simulink model "RobotX_ss_acousticsSKIP_dock_odoa_refer_model1021"  (R2014a)
settings: Solver=FixedStepDiscrete  StartTime=0.0  StopTime=inf  FixedStep=.25  RelTol=1e-3
undefined symbols (not defined in the file): Com1, Com2, Com3, Com4, DiscIntNeverNeededParam, standard
libraries: xpcseriallib x42, slrtlib x8, simulink x7, speedgoatlib x2, speedgoatlib_IO102 x1
(part 7 of 18)

== matlab function RobotX_ss_acousticsSKIP_dock_odoa_refer_model1021/Main FSM/ODOA/SLAM1/Models for prediction/Model7/Dynamic Model ==
  data: F_surge input; F_sway input; Torque input; u input; surgeAccel output; v input; psi input; swayAccel output; yawAccel output
function [surgeAccel, swayAccel, yawAccel] = ...
    WAM_V_3DOF(F_surge, F_sway, Torque, u, v, psi)
%Written by Anderson Lebbad on August 12, 2014
%Last Edited:

%This function was heavily based off of Ariel Qu's Vel3DOF_IvanV1. It was
%rewritten for real-time use.

%This function will produce the transient output surge velocity of a
%linearized model of the USV. It is assumed that the vehicle is equivalent
%to two cylinders in the water.

%%%%%DEFINED VARIABLE%%%%%%
%
%   Xext = Thrust from motors
%   Next = Moment from motor
%   m = Mass of vehicle
%   Xudot = Added mass in surge direction
%   Yvdot = Added mass in sway direction
%   Nrdot = Added mass from yaw
%   xg = offset from center of gravity
%   rho = density of seawater
%   S = wetted surface area
%   R = Reynolds number
%   Cd = Coefficient of drag
%   Cdc = Coefficient of drag for sway
%   nu = Kinematic viscosity
%   L = Length overall
%   T = draft
%   B = beam
%   SA = Surface area of cylinder experiencing sway
%   Iz = moment of inertia about Z axis
%
%%%%%%

% Force/Mometns from thrusters & control surfaces...

tau = [F_surge; F_sway; Torque];

% Calculate yaw rate
persistent lastHeading
if isempty(lastHeading)
    lastHeading = psi;
end
%Sample time
ts = .1;

r = (psi - lastHeading)/ts;

% Velocity & Angular velocity vectors
vel = [u; v; 0];
omega = [0; 0; r];

%define variables
m = 145.7;         % Total mass [kg] - reduced from 102
rho = 1025.9;   % density of seawater [kg/m^3]
L = 3.91*0.85;  % Length on the waterline [m]
B = 0.426;       % Demihull beam [m]
T = B*0.2;        % Draft of the demihull [m]
p_bar = 1.0; % sidehull separation - from centerplane vessel to centerplane demihull
Iz = 262.181;    % Mass moment of inertia about z-axis [kg*m^2]
xg = 0;         % Body-Fixed coordinate system taken to be center of gravity
yg = 0;         % Symmetrical Vessel
Cd = 1.1;       % Drag coefficient for a lateral cylinder
LCG = 1.485;        % Need to know where LCG wrt stern

% Vector location of port and starboard hulls
r_port = [-LCG; -p_bar; 0];   
r_stbd = [-LCG; p_bar; 0];

% Port and starboard hull velocities
vel_port = vel + cross(omega,r_port);
vel_stbd = vel + cross(omega,r_stbd);

u_port = vel_port(1);
u_stbd = vel_stbd(1);

% Port and starboard state vectors
state_port = vel_port + omega;
state_stbd = vel_stbd + omega;

%% Added Mass
% Estimated for each hull, then multiplied by 2 to account for both hulls
Xudot = -0.05*m;

%Using strip theory to estimate added mass coefficients
Nrdot = -(4.75/2*pi*rho*p_bar*T^4 + pi*rho*T^2*((L - LCG)^3 + LCG^3)/3);
Nvdot = - pi*rho*T^2*((L - LCG)^2 - LCG^2)/2;

Yrdot = Nvdot;
Yvdot = -rho*pi*T^2*L;

% Multiply by 2:
Xudot = 2*Xudot;
Nrdot = 2*Nrdot;
Nvdot = 2*Nvdot;
Yrdot = 2*Yrdot;
Yvdot = 2*Yvdot;

%Calculate Coefficient of Drag for Sway from 1950 SNAME approximation
Cdc= 1.1 + 0.0045*L/T - 0.1*B/T + 0.016*(B/T)^2;
SA = 2*pi/4*T*L; %projected area of pontoon for two pontoons

%% Linear Drag Terms
%Total Speed
U = sqrt(u^2+v^2);

Xu = 0;
Yv = -0.5*rho*abs(v)*2*Cdc*SA; %20 was the last working number %from SNAME 1950, x2 for two cylinders
%Nr = -0.5*pi*rho*U*T^2*L^2;
Nr = -pi*rho*U*T^2*L^2*.065;
Nv = -pi*rho*U*T^2*L*.01;
Yr = pi*rho*U*T^2*L*0.2;  %from Newman approximation in Lewandowski

%% Nonlinear Drag Terms

% Drag and Moment due to drag on entire vessel - includes nonlinear and
% linear drag terms
D_port = 0.5*(0.44*u_port^3 - 0.01*u_port^2 + 19*u_port);     % Can assume that this equation also takes into account Xu - so set Xu=0
D_stbd = 0.5*(0.44*u_stbd^3 - 0.01*u_stbd^2 + 19*u_stbd);     % Can assume that this equation also takes into account Xu - so set Xu=0

tau_drag = [-(D_port + D_stbd); 0; (D_stbd - D_port)*p_bar];

Xuu = 0;

%% Maneuvering Coefficient Matrices
% Added Mass Matrix
M = [(m - Xudot)      0              0;...
    0               (m - Yvdot)     (m*xg - Yrdot);...
    0               (m*xg - Nvdot)  (Iz - Nrdot)];

%Centripetal and Added Mass Centripetal force matrices
% C_RB = [
%     0                  0                0
%     0                  0                0
%     0                  0                0
%     ];

% C_RB = [
%     0                  0                -m*(xg*r + v)
%     0                  0                -m*(yg*r - u)
%     m*(xg*r + v)       m*(yg*r - u)     0
%     ];

% C_A = -[ %negative originally
%     0                               0           0
%     0                               0           0
%     0                               0           0
%     ];

% Negating centripetal acceleration for test
C_RB = 0;
C_A = 0;

D = -[Xu  0   0;...
      0   Yv  Yr;...
      0   Nv  Nr];

% Nonlinear Drag Coefficients
D_N = -[Xuu*u   0                       0;...
        0       0                       0;...
        0       0                       0];
    
%% Calculate the port and starboard force vectors
tau_port = -(C_RB + C_A + D + D_N)*state_port;
tau_stbd = -(C_RB + C_A + D + D_N)*state_stbd;


%% Sum the force vectors
tau_tot = tau + tau_drag + tau_port + tau_stbd...
    + cross(r_port,[tau_port(1);tau_port(2);0]) + ...
    cross(r_stbd,[tau_stbd(1);tau_stbd(2);0]);

% Calculate the time derivative of the state vector

accel = M\tau_tot;

%% Separate output

surgeAccel = accel(1);
swayAccel = accel(2);
yawAccel = accel(3);

end

== matlab function RobotX_ss_acousticsSKIP_dock_odoa_refer_model1021/Main FSM/ODOA/Path/LLA to NED ==
  data: LLAs input; NEDout output; NED_origin input
function NEDout = LLA2NEDfun(LLAs,NED_origin)
%Written by Anderson Lebbad on September 20, 2014
%Last edited by:
%
%This function converts a target Latitude, Longitude, Altitude (LLA) point
%into North, East, Down (NED) coordinates

NED  = zeros(4,2);
for i=1:4
%First convert to earth centered, earth fixed frame
GoalECEF = lla2ecef([LLAs(i,:)*(pi/180), 0]');
%Then convert from ECEF to North East Down
GoalNEDvect = ecef2ned(NED_origin'*(pi/180),GoalECEF);
NED(i,:) = GoalNEDvect(1:2)';
end


%Order outputs for grid
Xord = sortrows(NED,1);
Yord = sortrows(NED,2);

BLfirst = ismember(Yord(3:4,:),Xord(3,:),'rows');
if sum(BLfirst) >= 1
    BL = Xord(3,:);
    BR = Xord(4,:);
else
    BL = Xord(4,:);
    BR = Xord(3,:);
end

TRthird = ismember(Yord(1:2,:),Xord(1,:),'rows');
if sum(TRthird) >= 1
    TR = Xord(1,:);
    TL = Xord(2,:);
else
    TR = Xord(2,:);
    TL = Xord(1,:);
end

NEDout = [BL; BR; TL; TR];

end

function x_ecef = lla2ecef(x_lla)
% LLE2ECEF: Converts from geodetic latitude, longitude, and altitude to earth-centered earth-fixed Cartesian coordinates
% INPUT: latitude phi (rad), longitude lambda (rad), altitude h (m)
% OUTPUT: [x, y, z]' (m) earth-centered earth-fixed Cartesian coordinates
    a = 6378137; % equatorial radius of ellipsoid (semi-major axis) (m)
    b = 6356752; % polar axis radius of ellipsoid (semi-minor axis) (m)

    phi = x_lla(1);
    lambda = x_lla(2);
    h = x_lla(3);
    
    % auxiliar quantities f, e, and N
    f = (a-b)/a;
    e = f*(2-f);
    N = a/sqrt(1-(e*sin(phi))^2);
    x_ecef = [(N+h)*cos(phi)*cos(lambda); (N+h)*cos(phi)*sin(lambda); (N*(1-e^2)+h)*sin(phi)];
end

function [x_ned] = ecef2ned(ned_lla, x_ecef)
% ECEF2NED Converts from earth-centered, earth-fixed Cartesian coordinates to tangent plane
% INPUT:
% 1) x_ecef=[x,y,z]' (m) earth-centered, earth-fixed Cartesian coordinates
% 2) ned_lla=[phi,lambda]' consiting of latitude phi (rad), longitude lambda (rad) of NED origin
% OUTPUT:
% 1) x_ned=[x,y,z]' (m) in NED coordinate system with the origin [phi,lambda]'

    phi = ned_lla(1);
    lambda = ned_lla(2);

    % transformation  matrix
    T = [-sin(phi)*cos(lambda) -sin(phi)*sin(lambda)  cos(phi)
         -sin(lambda)           cos(lambda)           0
          cos(phi)*cos(lambda)   cos(phi)*sin(lambda)  sin(phi)];

     x_ned = T*(x_ecef-lla2ecef([phi, lambda, 0]')); % convert to NED
     x_ned(3) = -x_ned(3);
end

== matlab function RobotX_ss_acousticsSKIP_dock_odoa_refer_model1021/Main FSM/ODOA/SLAM1/Models for prediction/Model1/Stbd Thruster Model ==
  data: stbdMP input; F_surge output; stbdAzimuth input; F_sway output; Torque output
function [F_surge,F_sway,Torque]  = StarBoardThruster(stbdMP,stbdAzimuth)
%Approximation for Starboard Force and Moment with the input motor power
%and azimuth angle of thruster

%Longitudinal distance from center of mass
longDist =1.007;           %m

%Axial distance from center of mass
axialDist=1.485;            %m

%% Piece-wise thrust calculation

if stbdMP <= -51.0119
    F = .9140*stbdMP + 40;
elseif stbdMP >= 26.8367
    F = 1.658*stbdMP - 41.01;
else
    F = .12987*stbdMP;
end

%% Force components
F_surge=F*cos(stbdAzimuth*pi/180);       %N
F_sway=F*sin(stbdAzimuth*pi/180);       %N

%% Torque calculation

Torque = -F_surge*longDist - F_sway*axialDist;   %N.m

end

== system RobotX_ss_acousticsSKIP_dock_odoa_refer_model1021/Main FSM/ODOA/GPS Move/Output Reassign ==
  Vaild : Inport
  Data : Inport  Port=2
  Sensors : Inport  Port=3
  Acoustic Active : Constant  Value=0
  Bus Creator2 : BusCreator  Inputs=3
  Bus Creator3 : BusCreator  Inputs=3
  Bus Creator5 : BusCreator  Inputs=2
  Constant3 : Constant  Value=0
  Lidar Mode : Constant  Value=0
  Outputs : Outport
  wires:
  Sensors/1 -> Bus Creator5/2  "Sensors"
  Bus Creator5/1 -> Outputs/1  "Output Signals"
  Vaild/1 -> Bus Creator2/1  "Valid"
  Constant3/1 -> Bus Creator2/2  "Control Mode"
  Data/1 -> Bus Creator2/3  "Data"
  Bus Creator2/1 -> Bus Creator3/1  "Navigation Outputs"
  Acoustic Active/1 -> Bus Creator3/2  "Acoustic Active"
  Lidar Mode/1 -> Bus Creator3/3  "Lidar Mode"
  Bus Creator3/1 -> Bus Creator5/1  "Outputs"

== system RobotX_ss_acousticsSKIP_dock_odoa_refer_model1021/Main FSM/ODOA/Path/Output Reassign ==
  Vaild : Inport
  Data : Inport  Port=2
  Sensors : Inport  Port=3
  Acoustic Active : Constant  Value=0
  Bus Creator2 : BusCreator  Inputs=3
  Bus Creator3 : BusCreator  Inputs=3
  Bus Creator5 : BusCreator  Inputs=2
  Constant3 : Constant  Value=0
  Lidar Mode : Constant  Value=0
  Outputs : Outport
  wires:
  Sensors/1 -> Bus Creator5/2  "Sensors"
  Bus Creator5/1 -> Outputs/1  "Output Signals"
  Vaild/1 -> Bus Creator2/1  "Valid"
  Constant3/1 -> Bus Creator2/2  "Control Mode"
  Data/1 -> Bus Creator2/3  "Data"
  Bus Creator2/1 -> Bus Creator3/1  "Navigation Outputs"
  Acoustic Active/1 -> Bus Creator3/2  "Acoustic Active"
  Lidar Mode/1 -> Bus Creator3/3  "Lidar Mode"
  Bus Creator3/1 -> Bus Creator5/1  "Outputs"

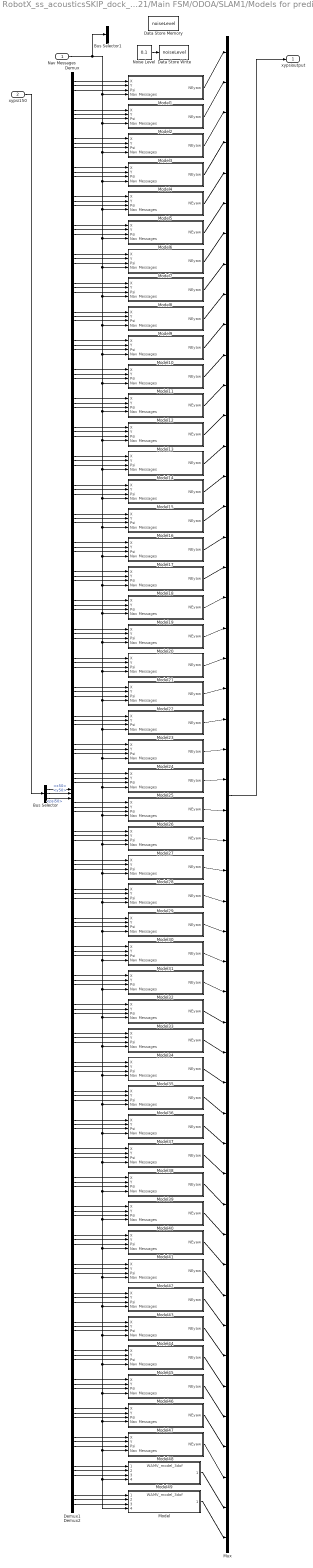
== system RobotX_ss_acousticsSKIP_dock_odoa_refer_model1021/Main FSM/ODOA/SLAM1/Models for prediction ==
  Nav Messages : Inport
  xypsi150 : Inport  Port=2
  Bus Selector : BusSelector  OutputSignals=x50,y50,psi50
  Bus Selector1 : BusSelector  OutputSignals=signal1,signal2
  Data Store Memory : DataStoreMemory  DataStoreName=noiseLevel  ReadBeforeWriteMsg=warning  WriteAfterWriteMsg=warning  WriteAfterReadMsg=warning
  Data Store Write : DataStoreWrite  DataStoreName=noiseLevel
  Demux : Demux  Outputs=50
  Demux1 : Demux  Outputs=50
  Demux2 : Demux  Outputs=50
  Model : ModelReference  ModelNameDialog=WAMV_model_3dof.slx  SimulationMode=Normal  ModelReferenceVersion=1.1919  CopyOfModelName=WAMV_model_3dof.slx  DefaultDataLogging=on
  Model1 : Subsystem
  Model10 : Subsystem
  Model11 : Subsystem
  Model12 : Subsystem
  Model13 : Subsystem
  Model14 : Subsystem
  Model15 : Subsystem
  Model16 : Subsystem
  Model17 : Subsystem
  Model18 : Subsystem
  Model19 : Subsystem
  Model2 : Subsystem
  Model20 : Subsystem
  Model21 : Subsystem
  Model22 : Subsystem
  Model23 : Subsystem
  Model24 : Subsystem
  Model25 : Subsystem
  Model26 : Subsystem
  Model27 : Subsystem
  Model28 : Subsystem
  Model29 : Subsystem
  Model3 : Subsystem
  Model30 : Subsystem
  Model31 : Subsystem
  Model32 : Subsystem
  Model33 : Subsystem
  Model34 : Subsystem
  Model35 : Subsystem
  Model36 : Subsystem
  Model37 : Subsystem
  Model38 : Subsystem
  Model39 : Subsystem
  Model4 : Subsystem
  Model40 : Subsystem
  Model41 : Subsystem
  Model42 : Subsystem
  Model43 : Subsystem
  Model44 : Subsystem
  Model45 : Subsystem
  Model46 : Subsystem
  Model47 : Subsystem
  Model48 : Subsystem
  Model49 : ModelReference  ModelNameDialog=WAMV_model_3dof.slx  SimulationMode=Normal  ModelReferenceVersion=1.1919  CopyOfModelName=WAMV_model_3dof.slx  DefaultDataLogging=on
  Model5 : Subsystem
  Model6 : Subsystem
  Model7 : Subsystem
  Model8 : Subsystem
  Model9 : Subsystem
  Mux : Mux  Inputs=50
  Noise Level : Constant  Value=0.1
  xypsioutput : Outport  PortDimensions=150
  wires:
  Noise Level/1 -> Data Store Write/1
  Demux/1 -> Model1/1(X)
  Demux1/1 -> Model1/2(Y)
  Demux2/1 -> Model1/3(Psi)
  Demux/2 -> Model2/1(X)
  Demux1/2 -> Model2/2(Y)
  Demux2/2 -> Model2/3(Psi)
  Demux/3 -> Model3/1(X)
  Demux1/3 -> Model3/2(Y)
  Demux2/3 -> Model3/3(Psi)
  Demux/4 -> Model4/1(X)
  Demux1/4 -> Model4/2(Y)
  Demux2/4 -> Model4/3(Psi)
  Demux/5 -> Model5/1(X)
  Demux1/5 -> Model5/2(Y)
  Demux2/5 -> Model5/3(Psi)
  Demux/6 -> Model6/1(X)
  Demux1/6 -> Model6/2(Y)
  Demux2/6 -> Model6/3(Psi)
  Nav Messages/1 -> Bus Selector1/1, Model1/4(Nav Messages), Model2/4(Nav Messages), Model3/4(Nav Messages), Model4/4(Nav Messages), Model5/4(Nav Messages), Model6/4(Nav Messages), Model7/4(Nav Messages), Model8/4(Nav Messages), Model9/4(Nav Messages), Model10/4(Nav Messages), Model11/4(Nav Messages), Model12/4(Nav Messages), Model13/4(Nav Messages), Model14/4(Nav Messages), Model15/4(Nav Messages), Model16/4(Nav Messages), Model17/4(Nav Messages), Model18/4(Nav Messages), Model19/4(Nav Messages), Model20/4(Nav Messages), Model21/4(Nav Messages), Model22/4(Nav Messages), Model23/4(Nav Messages), Model24/4(Nav Messages), Model25/4(Nav Messages), Model26/4(Nav Messages), Model27/4(Nav Messages), Model28/4(Nav Messages), Model29/4(Nav Messages), Model30/4(Nav Messages), Model31/4(Nav Messages), Model32/4(Nav Messages), Model33/4(Nav Messages), Model34/4(Nav Messages), Model35/4(Nav Messages), Model36/4(Nav Messages), Model37/4(Nav Messages), Model38/4(Nav Messages), Model39/4(Nav Messages), Model40/4(Nav Messages), Model41/4(Nav Messages), Model42/4(Nav Messages), Model43/4(Nav Messages), Model44/4(Nav Messages), Model45/4(Nav Messages), Model46/4(Nav Messages), Model47/4(Nav Messages), Model48/4(Nav Messages), Model49/4, Model/4
  Demux2/15 -> Model15/3(Psi)
  Demux1/15 -> Model15/2(Y)
  Demux/15 -> Model15/1(X)
  Demux2/14 -> Model14/3(Psi)
  Demux1/14 -> Model14/2(Y)
  Demux/14 -> Model14/1(X)
  Demux2/13 -> Model13/3(Psi)
  Demux1/13 -> Model13/2(Y)
  Demux/13 -> Model13/1(X)
  Demux2/12 -> Model12/3(Psi)
  Demux1/12 -> Model12/2(Y)
  Demux/12 -> Model12/1(X)
  Demux2/11 -> Model11/3(Psi)
  Demux1/11 -> Model11/2(Y)
  Demux/11 -> Model11/1(X)
  Demux2/10 -> Model10/3(Psi)
  Demux1/10 -> Model10/2(Y)
  Demux/10 -> Model10/1(X)
  Demux2/9 -> Model9/3(Psi)
  Demux1/9 -> Model9/2(Y)
  Demux/9 -> Model9/1(X)
  Demux2/8 -> Model8/3(Psi)
  Demux1/8 -> Model8/2(Y)
  Demux/8 -> Model8/1(X)
  Demux2/7 -> Model7/3(Psi)
  Demux1/7 -> Model7/2(Y)
  Demux/7 -> Model7/1(X)
  Demux/16 -> Model16/1(X)
  Demux1/16 -> Model16/2(Y)
  Demux2/16 -> Model16/3(Psi)
  Demux/17 -> Model17/1(X)
  Demux1/17 -> Model17/2(Y)
  Demux2/17 -> Model17/3(Psi)
  Demux/18 -> Model18/1(X)
  Demux1/18 -> Model18/2(Y)
  Demux2/18 -> Model18/3(Psi)
  Demux/19 -> Model19/1(X)
  Demux1/19 -> Model19/2(Y)
  Demux2/19 -> Model19/3(Psi)
  Demux/20 -> Model20/1(X)
  Demux1/20 -> Model20/2(Y)
  Demux2/20 -> Model20/3(Psi)
  Demux/21 -> Model21/1(X)
  Demux1/21 -> Model21/2(Y)
  Demux2/21 -> Model21/3(Psi)
  Demux/22 -> Model22/1(X)
  Demux1/22 -> Model22/2(Y)
  Demux2/22 -> Model22/3(Psi)
  Demux/23 -> Model23/1(X)
  Demux1/23 -> Model23/2(Y)
  Demux2/23 -> Model23/3(Psi)
  Demux/24 -> Model24/1(X)
  Demux1/24 -> Model24/2(Y)
  Demux2/24 -> Model24/3(Psi)
  Demux/25 -> Model25/1(X)
  Demux1/25 -> Model25/2(Y)
  Demux2/25 -> Model25/3(Psi)
  Demux/26 -> Model26/1(X)
  Demux1/26 -> Model26/2(Y)
  Demux2/26 -> Model26/3(Psi)
  Demux/27 -> Model27/1(X)
  Demux1/27 -> Model27/2(Y)
  Demux2/27 -> Model27/3(Psi)
  Demux/28 -> Model28/1(X)
  Demux1/28 -> Model28/2(Y)
  Demux2/28 -> Model28/3(Psi)
  Demux/29 -> Model29/1(X)
  Demux1/29 -> Model29/2(Y)
  Demux2/29 -> Model29/3(Psi)
  Demux/30 -> Model30/1(X)
  Demux1/30 -> Model30/2(Y)
  Demux2/30 -> Model30/3(Psi)
  Demux/31 -> Model31/1(X)
  Demux1/31 -> Model31/2(Y)
  Demux2/31 -> Model31/3(Psi)
  Demux/32 -> Model32/1(X)
  Demux1/32 -> Model32/2(Y)
  Demux2/32 -> Model32/3(Psi)
  Demux/33 -> Model33/1(X)
  Demux1/33 -> Model33/2(Y)
  Demux2/33 -> Model33/3(Psi)
  Demux/34 -> Model34/1(X)
  Demux1/34 -> Model34/2(Y)
  Demux2/34 -> Model34/3(Psi)
  Demux/35 -> Model35/1(X)
  Demux1/35 -> Model35/2(Y)
  Demux2/35 -> Model35/3(Psi)
  Demux/36 -> Model36/1(X)
  Demux1/36 -> Model36/2(Y)
  Demux2/36 -> Model36/3(Psi)
  Demux/37 -> Model37/1(X)
  Demux1/37 -> Model37/2(Y)
  Demux2/37 -> Model37/3(Psi)
  Demux/38 -> Model38/1(X)
  Demux1/38 -> Model38/2(Y)
  Demux2/38 -> Model38/3(Psi)
  Demux/39 -> Model39/1(X)
  Demux1/39 -> Model39/2(Y)
  Demux2/39 -> Model39/3(Psi)
  Demux/40 -> Model40/1(X)
  Demux1/40 -> Model40/2(Y)
  Demux2/40 -> Model40/3(Psi)
  Demux/41 -> Model41/1(X)
  Demux1/41 -> Model41/2(Y)
  Demux2/41 -> Model41/3(Psi)
  Demux/42 -> Model42/1(X)
  Demux1/42 -> Model42/2(Y)
  Demux2/42 -> Model42/3(Psi)
  Demux/43 -> Model43/1(X)
  Demux1/43 -> Model43/2(Y)
  Demux2/43 -> Model43/3(Psi)
  Demux/44 -> Model44/1(X)
  Demux1/44 -> Model44/2(Y)
  Demux2/44 -> Model44/3(Psi)
  Demux/45 -> Model45/1(X)
  Demux1/45 -> Model45/2(Y)
  Demux2/45 -> Model45/3(Psi)
  Demux/46 -> Model46/1(X)
  Demux1/46 -> Model46/2(Y)
  Demux2/46 -> Model46/3(Psi)
  Demux/47 -> Model47/1(X)
  Demux1/47 -> Model47/2(Y)
  Demux2/47 -> Model47/3(Psi)
  Demux/48 -> Model48/1(X)
  Demux1/48 -> Model48/2(Y)
  Demux2/48 -> Model48/3(Psi)
  Demux/49 -> Model49/1
  Demux1/49 -> Model49/2
  Demux2/49 -> Model49/3
  Demux/50 -> Model/1
  Demux1/50 -> Model/2
  Demux2/50 -> Model/3
  xypsi150/1 -> Bus Selector/1
  Bus Selector/1 -> Demux/1  "<x50>"
  Bus Selector/2 -> Demux1/1  "<y50>"
  Bus Selector/3 -> Demux2/1  "<psi50>"
  Model27/1(NEyaw) -> Mux/27
  Model26/1(NEyaw) -> Mux/26
  Model25/1(NEyaw) -> Mux/25
  Model24/1(NEyaw) -> Mux/24
  Model28/1(NEyaw) -> Mux/28
  Model23/1(NEyaw) -> Mux/23
  Model21/1(NEyaw) -> Mux/21
  Model30/1(NEyaw) -> Mux/30
  Model29/1(NEyaw) -> Mux/29
  Model22/1(NEyaw) -> Mux/22
  Model40/1(NEyaw) -> Mux/40
  Model33/1(NEyaw) -> Mux/33
  Model36/1(NEyaw) -> Mux/36
  Model38/1(NEyaw) -> Mux/38
  Model37/1(NEyaw) -> Mux/37
  Model35/1(NEyaw) -> Mux/35
  Model39/1(NEyaw) -> Mux/39
  Model31/1(NEyaw) -> Mux/31
  Model32/1(NEyaw) -> Mux/32
  Model34/1(NEyaw) -> Mux/34
  Model2/1(NEyaw) -> Mux/2
  Model5/1(NEyaw) -> Mux/5
  Model3/1(NEyaw) -> Mux/3
  Model4/1(NEyaw) -> Mux/4
  Model19/1(NEyaw) -> Mux/19
  Model13/1(NEyaw) -> Mux/13
  Model14/1(NEyaw) -> Mux/14
  Model12/1(NEyaw) -> Mux/12
  Model16/1(NEyaw) -> Mux/16
  Model17/1(NEyaw) -> Mux/17
  Model18/1(NEyaw) -> Mux/18
  Model20/1(NEyaw) -> Mux/20
  Model11/1(NEyaw) -> Mux/11
  Model15/1(NEyaw) -> Mux/15
  Model10/1(NEyaw) -> Mux/10
  Model8/1(NEyaw) -> Mux/8
  Model9/1(NEyaw) -> Mux/9
  Model7/1(NEyaw) -> Mux/7
  Model6/1(NEyaw) -> Mux/6
  Model48/1(NEyaw) -> Mux/48
  Model42/1(NEyaw) -> Mux/42
  Model49/1 -> Mux/49
  Model47/1(NEyaw) -> Mux/47
  Model/1 -> Mux/50
  Model43/1(NEyaw) -> Mux/43
  Model45/1(NEyaw) -> Mux/45
  Model44/1(NEyaw) -> Mux/44
  Model46/1(NEyaw) -> Mux/46
  Model41/1(NEyaw) -> Mux/41
  Model1/1(NEyaw) -> Mux/1
  Mux/1 -> xypsioutput/1

== system RobotX_ss_acousticsSKIP_dock_odoa_refer_model1021/Main FSM/ODOA/SLAM1/SLAM enabled ==
  pre_past_positions : Inport
  lm_data : Inport  Port=2
  positionboat : Inport  Port=3
  Enable : EnablePort
  slammed : MATLAB Function  TreatAsAtomicUnit=on
  mpa : Outport
  part_positions : Outport  Port=2
  wires:
  lm_data/1 -> slammed/1(lm_data)
  pre_past_positions/1 -> slammed/2(pre_part_positions)
  slammed/1(mpa) -> mpa/1
  slammed/2(part_positions) -> part_positions/1
  positionboat/1 -> slammed/3(positionboat)

== system RobotX_ss_acousticsSKIP_dock_odoa_refer_model1021/Main FSM/ODOA/SLAM1/inputselection ==
  controlchange : Inport
  xypsi : Inport  Port=2
  Landmarkchange : Inport  Port=3
  part_positions : Inport  Port=4
  xypsi150 : Inport  Port=5
  Bus Creator : BusCreator  Inputs=3
  Delay{,1..4} (5 alike) : Delay  DelayLength=1  InitialCondition=0
  MATLAB Function : MATLAB Function  TreatAsAtomicUnit=on
  last particle positions : Outport
  wires:
  Delay/1 -> MATLAB Function/4(part_positions)
  Delay1/1 -> MATLAB Function/3(xypsi)
  Delay2/1 -> MATLAB Function/5(xypsi150)
  Delay4/1 -> MATLAB Function/1(Landmarkchange)
  Delay3/1 -> MATLAB Function/2(controlchange)
  controlchange/1 -> Delay3/1
  xypsi/1 -> Delay1/1
  part_positions/1 -> Delay/1
  Landmarkchange/1 -> Delay4/1
  xypsi150/1 -> Delay2/1
  MATLAB Function/2(y50) -> Bus Creator/2  "y50"
  MATLAB Function/3(psi50) -> Bus Creator/3  "psi50"
  MATLAB Function/1(x50) -> Bus Creator/1  "x50"
  Bus Creator/1 -> last particle positions/1  "last particle positions"

== system RobotX_ss_acousticsSKIP_dock_odoa_refer_model1021/Main FSM/Start//Speedgate/Aim/Output Heirarchy ==
  Data : Inport
  Sensors : Inport  Port=2
  Acoustic Active : Constant  Value=0
  Bus Creator2 : BusCreator  Inputs=3
  Bus Creator3 : BusCreator  Inputs=3
  Bus Creator5 : BusCreator  Inputs=2
  Constant : Constant
  Constant3 : Constant
  Lidar Mode : Constant
  Outputs : Outport
  wires:
  Sensors/1 -> Bus Creator5/2  "Sensors"
  Bus Creator5/1 -> Outputs/1  "Output Signals"
  Constant/1 -> Bus Creator2/1  "Valid"
  Constant3/1 -> Bus Creator2/2  "Control Mode"
  Data/1 -> Bus Creator2/3  "Data"
  Bus Creator2/1 -> Bus Creator3/1  "Navigation Outputs"
  Acoustic Active/1 -> Bus Creator3/2  "Acoustic Active"
  Lidar Mode/1 -> Bus Creator3/3  "Lidar Mode"
  Bus Creator3/1 -> Bus Creator5/1  "Outputs"

== system RobotX_ss_acousticsSKIP_dock_odoa_refer_model1021/Main FSM/Start//Speedgate/Dead Reckon/Output Reassign ==
  Vaild : Inport
  Data : Inport  Port=2
  Sensors : Inport  Port=3
  Acoustic Active : Constant  Value=0
  Bus Creator2 : BusCreator  Inputs=3
  Bus Creator3 : BusCreator  Inputs=3
  Bus Creator5 : BusCreator  Inputs=2
  Constant3 : Constant  Value=0
  Lidar Mode : Constant  Value=3
  Outputs : Outport
  wires:
  Sensors/1 -> Bus Creator5/2  "Sensors"
  Bus Creator5/1 -> Outputs/1  "Output Signals"
  Vaild/1 -> Bus Creator2/1  "Valid"
  Constant3/1 -> Bus Creator2/2  "Control Mode"
  Data/1 -> Bus Creator2/3  "Data"
  Bus Creator2/1 -> Bus Creator3/1  "Navigation Outputs"
  Acoustic Active/1 -> Bus Creator3/2  "Acoustic Active"
  Lidar Mode/1 -> Bus Creator3/3  "Lidar Mode"
  Bus Creator3/1 -> Bus Creator5/1  "Outputs"

== system RobotX_ss_acousticsSKIP_dock_odoa_refer_model1021/Main FSM/Start//Speedgate/GPS Move/Output Reassign ==
  Vaild : Inport
  Data : Inport  Port=2
  Sensors : Inport  Port=3
  Acoustic Active : Constant  Value=0
  Bus Creator2 : BusCreator  Inputs=3
  Bus Creator3 : BusCreator  Inputs=3
  Bus Creator5 : BusCreator  Inputs=2
  Constant3 : Constant  Value=0
  Lidar Mode : Constant  Value=0
  Outputs : Outport
  wires:
  Sensors/1 -> Bus Creator5/2  "Sensors"
  Bus Creator5/1 -> Outputs/1  "Output Signals"
  Vaild/1 -> Bus Creator2/1  "Valid"
  Constant3/1 -> Bus Creator2/2  "Control Mode"
  Data/1 -> Bus Creator2/3  "Data"
  Bus Creator2/1 -> Bus Creator3/1  "Navigation Outputs"
  Acoustic Active/1 -> Bus Creator3/2  "Acoustic Active"
  Lidar Mode/1 -> Bus Creator3/3  "Lidar Mode"
  Bus Creator3/1 -> Bus Creator5/1  "Outputs"

== system RobotX_ss_acousticsSKIP_dock_odoa_refer_model1021/Sensors/1021 Comms/Message Selector/HRT Message ==
  Parameters : Inport
  Time : Inport  Port=2
  Bus Selector : BusSelector  OutputSignals=Sensors.Navigation Message.GPS (LLA).Lat,Sensors.Navigation Message.GPS (LLA).Long,Sensors.Navigation Message.On/Off/RC/Auto,Main Task
  MATLAB Function : MATLAB Function  TreatAsAtomicUnit=on
  HRT Message : Outport
  wires:
  MATLAB Function/1(asciiHRT) -> HRT Message/1
  Parameters/1 -> Bus Selector/1
  Time/1 -> MATLAB Function/1(Time)
  Bus Selector/1 -> MATLAB Function/2(HRTLat)  "<Lat>"
  Bus Selector/2 -> MATLAB Function/3(HRTLong)  "<Long>"
  Bus Selector/3 -> MATLAB Function/4(HRTMode)  "<On/Off/RC/Auto>"
  Bus Selector/4 -> MATLAB Function/5(HRTTask)  "<Main Task>"

== system RobotX_ss_acousticsSKIP_dock_odoa_refer_model1021/Sensors/1021 Comms/Message Selector/HRTLIT Message ==
  Parameters : Inport
  Time : Inport  Port=2
  Bus Selector : BusSelector  OutputSignals=Sensors.Navigation Message.GPS (LLA).Lat,Sensors.Navigation Message.GPS (LLA).Long,Main Task,Sensors.Navigation Message.On/Off/RC/Auto
  Data Store Read1 : DataStoreRead  DataStoreName=ltSeq
  MATLAB Function : MATLAB Function  TreatAsAtomicUnit=on
  MATLAB Function1 : MATLAB Function  TreatAsAtomicUnit=on
  HRTLIT Message : Outport
  wires:
  MATLAB Function/1(asciiHRTLIT) -> HRTLIT Message/1
  Time/1 -> MATLAB Function/1(Time)
  Parameters/1 -> Bus Selector/1
  Bus Selector/3 -> MATLAB Function/4(HRTTask)  "<Main Task>"
  Bus Selector/2 -> MATLAB Function/3(HRTLong)  "<Long>"
  Bus Selector/1 -> MATLAB Function/2(HRTLat)  "<Lat>"
  Bus Selector/4 -> MATLAB Function/5(HRTMode)  "<On/Off/RC/Auto>"
  Data Store Read1/1 -> MATLAB Function1/1(ltSeq)
  MATLAB Function1/2(LITSequence) -> MATLAB Function/7(LITSequence)
  MATLAB Function1/1(LITValid) -> MATLAB Function/6(LITValid)

== system RobotX_ss_acousticsSKIP_dock_odoa_refer_model1021/Sensors/1021 Comms/Message Selector/HRTSEA Message ==
  Parameters : Inport
  Time : Inport  Port=2
  Bus Selector : BusSelector  OutputSignals=Sensors.Navigation Message.GPS (LLA).Lat,Sensors.Navigation Message.GPS (LLA).Long,Main Task,Sensors.Navigation Message.On/Off/RC/Auto
  Data Store Read3 : DataStoreRead  DataStoreName=pingerInfo
  MATLAB Function : MATLAB Function  TreatAsAtomicUnit=on
  MATLAB Function1 : MATLAB Function  TreatAsAtomicUnit=on
  HRTSEA Message : Outport
  wires:
  MATLAB Function/1(asciiHRTSEA) -> HRTSEA Message/1
  Parameters/1 -> Bus Selector/1
  Time/1 -> MATLAB Function/1(Time)
  Data Store Read3/1 -> MATLAB Function1/1(pingerInfo)
  Bus Selector/3 -> MATLAB Function/4(HRTTask)  "<Main Task>"
  Bus Selector/1 -> MATLAB Function/2(HRTLat)  "<Lat>"
  Bus Selector/2 -> MATLAB Function/3(HRTLong)  "<Long>"
  Bus Selector/4 -> MATLAB Function/5(HRTMode)  "<On/Off/RC/Auto>"
  MATLAB Function1/3(SEALong) -> MATLAB Function/8(SEALong)
  MATLAB Function1/2(SEALat) -> MATLAB Function/7(SEALat)
  MATLAB Function1/5(SEADepth) -> MATLAB Function/10(SEADepth)
  MATLAB Function1/4(SEAColor) -> MATLAB Function/9(SEAColor)
  MATLAB Function1/1(SEAValid) -> MATLAB Function/6(SEAValid)

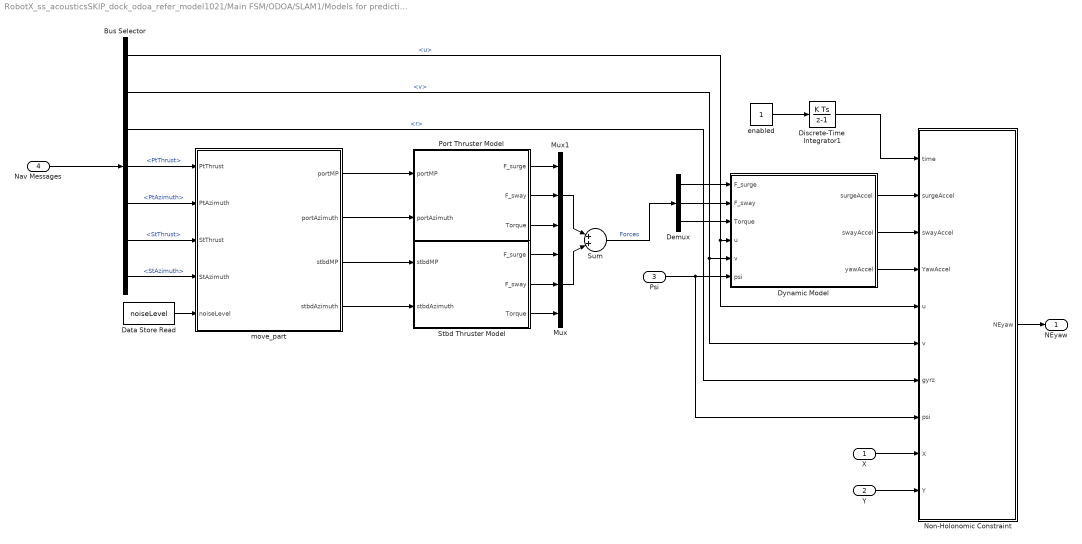
== system RobotX_ss_acousticsSKIP_dock_odoa_refer_model1021/Main FSM/ODOA/SLAM1/Models for prediction/Model1 ==
  X : Inport
  Y : Inport  Port=2
  Psi : Inport  Port=3
  Nav Messages : Inport  Port=4
  Bus Selector : BusSelector  OutputSignals=Velocity.u,Velocity.v,Velocity.r,Port.PtThrust,Port.PtAzimuth,Stbd.StThrust,Stbd.StAzimuth
  Data Store Read : DataStoreRead  DataStoreName=noiseLevel
  Demux : Demux  Outputs=3
  Discrete-Time Integrator1 : DiscreteIntegrator  SampleTime=-1  ICPrevOutput=DiscIntNeverNeededParam  ICPrevScaledInput=DiscIntNeverNeededParam
  Dynamic Model : MATLAB Function  TreatAsAtomicUnit=on
  Mux : Mux  Inputs=3
  Mux1 : Mux  Inputs=3
  Non-Holonomic Constraint : MATLAB Function  TreatAsAtomicUnit=on
  Port Thruster Model : MATLAB Function  TreatAsAtomicUnit=on
  Stbd Thruster Model : MATLAB Function  TreatAsAtomicUnit=on
  Sum : Sum  Inputs=|++|
  enabled : Constant
  move_part : MATLAB Function  TreatAsAtomicUnit=on
  NEyaw : Outport
  wires:
  Sum/1 -> Demux/1  "Forces"
  Bus Selector/2 -> Non-Holonomic Constraint/6(v), Dynamic Model/5(v)  "<v>"
  Bus Selector/1 -> Non-Holonomic Constraint/5(u), Dynamic Model/4(u)  "<u>"
  Psi/1 -> Non-Holonomic Constraint/8(psi), Dynamic Model/6(psi)
  Demux/2 -> Dynamic Model/2(F_sway)
  Demux/3 -> Dynamic Model/3(Torque)
  Demux/1 -> Dynamic Model/1(F_surge)
  Mux/1 -> Sum/2
  Stbd Thruster Model/1(F_surge) -> Mux/1
  Stbd Thruster Model/3(Torque) -> Mux/3
  Stbd Thruster Model/2(F_sway) -> Mux/2
  Mux1/1 -> Sum/1
  Port Thruster Model/2(F_sway) -> Mux1/2
  Port Thruster Model/1(F_surge) -> Mux1/1
  Port Thruster Model/3(Torque) -> Mux1/3
  Dynamic Model/1(surgeAccel) -> Non-Holonomic Constraint/2(surgeAccel)
  Dynamic Model/2(swayAccel) -> Non-Holonomic Constraint/3(swayAccel)
  Dynamic Model/3(yawAccel) -> Non-Holonomic Constraint/4(YawAccel)
  Y/1 -> Non-Holonomic Constraint/10(Y)
  X/1 -> Non-Holonomic Constraint/9(X)
  Bus Selector/3 -> Non-Holonomic Constraint/7(gyrz)  "<r>"
  Non-Holonomic Constraint/1(NEyaw) -> NEyaw/1
  enabled/1 -> Discrete-Time Integrator1/1
  Discrete-Time Integrator1/1 -> Non-Holonomic Constraint/1(time)
  Nav Messages/1 -> Bus Selector/1
  Bus Selector/4 -> move_part/1(PtThrust)  "<PtThrust>"
  Bus Selector/5 -> move_part/2(PtAzimuth)  "<PtAzimuth>"
  Bus Selector/7 -> move_part/4(StAzimuth)  "<StAzimuth>"
  Bus Selector/6 -> move_part/3(StThrust)  "<StThrust>"
  move_part/1(portMP) -> Port Thruster Model/1(portMP)
  move_part/2(portAzimuth) -> Port Thruster Model/2(portAzimuth)
  move_part/3(stbdMP) -> Stbd Thruster Model/1(stbdMP)
  move_part/4(stbdAzimuth) -> Stbd Thruster Model/2(stbdAzimuth)
  Data Store Read/1 -> move_part/5(noiseLevel)

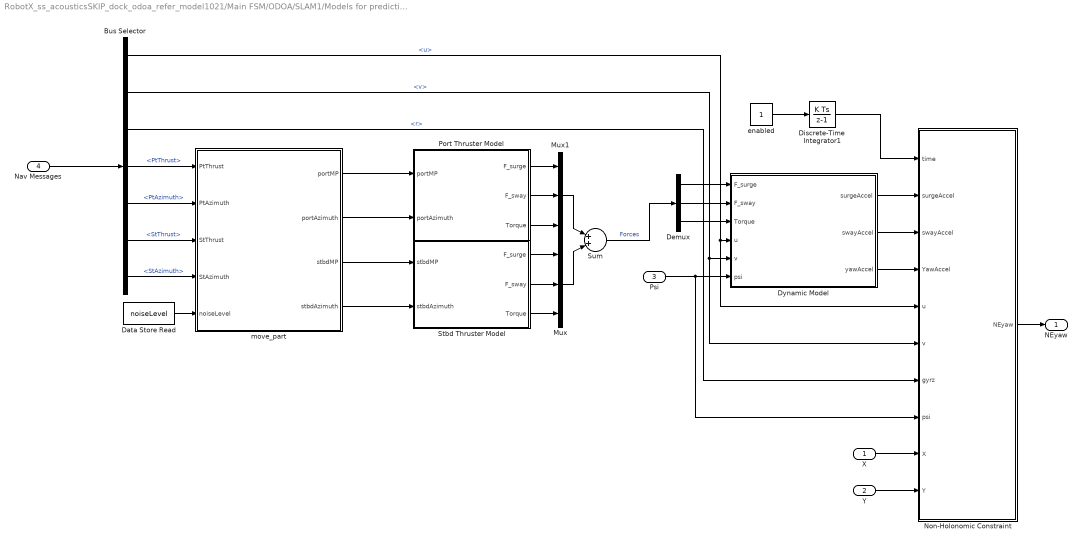
== system RobotX_ss_acousticsSKIP_dock_odoa_refer_model1021/Main FSM/ODOA/SLAM1/Models for prediction/Model10 ==
  X : Inport
  Y : Inport  Port=2
  Psi : Inport  Port=3
  Nav Messages : Inport  Port=4
  Bus Selector : BusSelector  OutputSignals=Velocity.u,Velocity.v,Velocity.r,Port.PtThrust,Port.PtAzimuth,Stbd.StThrust,Stbd.StAzimuth
  Data Store Read : DataStoreRead  DataStoreName=noiseLevel
  Demux : Demux  Outputs=3
  Discrete-Time Integrator1 : DiscreteIntegrator  SampleTime=-1  ICPrevOutput=DiscIntNeverNeededParam  ICPrevScaledInput=DiscIntNeverNeededParam
  Dynamic Model : MATLAB Function  TreatAsAtomicUnit=on
  Mux : Mux  Inputs=3
  Mux1 : Mux  Inputs=3
  Non-Holonomic Constraint : MATLAB Function  TreatAsAtomicUnit=on
  Port Thruster Model : MATLAB Function  TreatAsAtomicUnit=on
  Stbd Thruster Model : MATLAB Function  TreatAsAtomicUnit=on
  Sum : Sum  Inputs=|++|
  enabled : Constant
  move_part : MATLAB Function  TreatAsAtomicUnit=on
  NEyaw : Outport
  wires:
  Sum/1 -> Demux/1  "Forces"
  Bus Selector/2 -> Non-Holonomic Constraint/6(v), Dynamic Model/5(v)  "<v>"
  Bus Selector/1 -> Non-Holonomic Constraint/5(u), Dynamic Model/4(u)  "<u>"
  Psi/1 -> Non-Holonomic Constraint/8(psi), Dynamic Model/6(psi)
  Demux/2 -> Dynamic Model/2(F_sway)
  Demux/3 -> Dynamic Model/3(Torque)
  Demux/1 -> Dynamic Model/1(F_surge)
  Mux/1 -> Sum/2
  Stbd Thruster Model/1(F_surge) -> Mux/1
  Stbd Thruster Model/3(Torque) -> Mux/3
  Stbd Thruster Model/2(F_sway) -> Mux/2
  Mux1/1 -> Sum/1
  Port Thruster Model/2(F_sway) -> Mux1/2
  Port Thruster Model/1(F_surge) -> Mux1/1
  Port Thruster Model/3(Torque) -> Mux1/3
  Dynamic Model/1(surgeAccel) -> Non-Holonomic Constraint/2(surgeAccel)
  Dynamic Model/2(swayAccel) -> Non-Holonomic Constraint/3(swayAccel)
  Dynamic Model/3(yawAccel) -> Non-Holonomic Constraint/4(YawAccel)
  Y/1 -> Non-Holonomic Constraint/10(Y)
  X/1 -> Non-Holonomic Constraint/9(X)
  Bus Selector/3 -> Non-Holonomic Constraint/7(gyrz)  "<r>"
  Non-Holonomic Constraint/1(NEyaw) -> NEyaw/1
  enabled/1 -> Discrete-Time Integrator1/1
  Discrete-Time Integrator1/1 -> Non-Holonomic Constraint/1(time)
  Nav Messages/1 -> Bus Selector/1
  Bus Selector/4 -> move_part/1(PtThrust)  "<PtThrust>"
  Bus Selector/5 -> move_part/2(PtAzimuth)  "<PtAzimuth>"
  Bus Selector/7 -> move_part/4(StAzimuth)  "<StAzimuth>"
  Bus Selector/6 -> move_part/3(StThrust)  "<StThrust>"
  move_part/1(portMP) -> Port Thruster Model/1(portMP)
  move_part/2(portAzimuth) -> Port Thruster Model/2(portAzimuth)
  move_part/3(stbdMP) -> Stbd Thruster Model/1(stbdMP)
  move_part/4(stbdAzimuth) -> Stbd Thruster Model/2(stbdAzimuth)
  Data Store Read/1 -> move_part/5(noiseLevel)

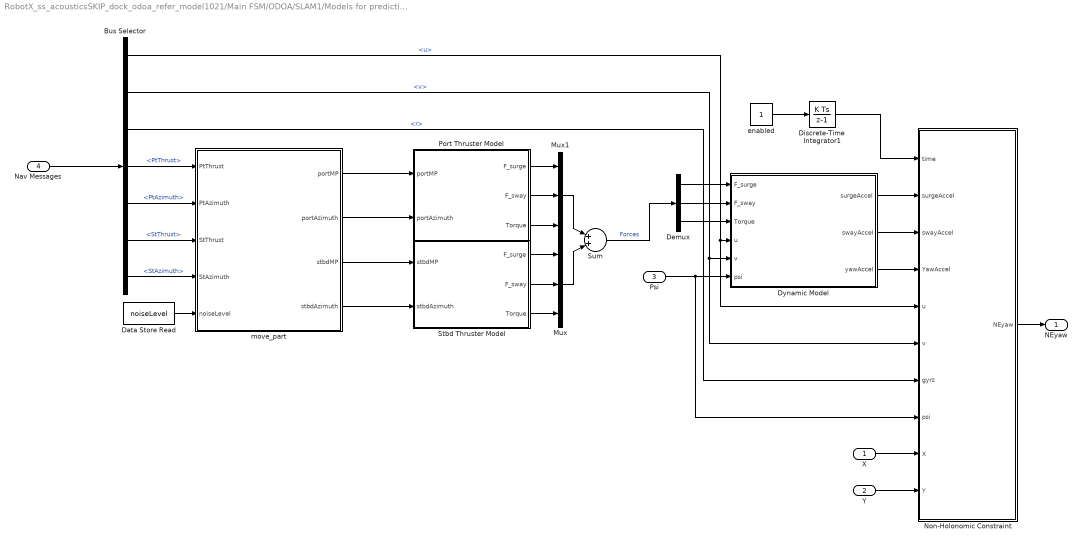
== system RobotX_ss_acousticsSKIP_dock_odoa_refer_model1021/Main FSM/ODOA/SLAM1/Models for prediction/Model11 ==
  X : Inport
  Y : Inport  Port=2
  Psi : Inport  Port=3
  Nav Messages : Inport  Port=4
  Bus Selector : BusSelector  OutputSignals=Velocity.u,Velocity.v,Velocity.r,Port.PtThrust,Port.PtAzimuth,Stbd.StThrust,Stbd.StAzimuth
  Data Store Read : DataStoreRead  DataStoreName=noiseLevel
  Demux : Demux  Outputs=3
  Discrete-Time Integrator1 : DiscreteIntegrator  SampleTime=-1  ICPrevOutput=DiscIntNeverNeededParam  ICPrevScaledInput=DiscIntNeverNeededParam
  Dynamic Model : MATLAB Function  TreatAsAtomicUnit=on
  Mux : Mux  Inputs=3
  Mux1 : Mux  Inputs=3
  Non-Holonomic Constraint : MATLAB Function  TreatAsAtomicUnit=on
  Port Thruster Model : MATLAB Function  TreatAsAtomicUnit=on
  Stbd Thruster Model : MATLAB Function  TreatAsAtomicUnit=on
  Sum : Sum  Inputs=|++|
  enabled : Constant
  move_part : MATLAB Function  TreatAsAtomicUnit=on
  NEyaw : Outport
  wires:
  Sum/1 -> Demux/1  "Forces"
  Bus Selector/2 -> Non-Holonomic Constraint/6(v), Dynamic Model/5(v)  "<v>"
  Bus Selector/1 -> Non-Holonomic Constraint/5(u), Dynamic Model/4(u)  "<u>"
  Psi/1 -> Non-Holonomic Constraint/8(psi), Dynamic Model/6(psi)
  Demux/2 -> Dynamic Model/2(F_sway)
  Demux/3 -> Dynamic Model/3(Torque)
  Demux/1 -> Dynamic Model/1(F_surge)
  Mux/1 -> Sum/2
  Stbd Thruster Model/1(F_surge) -> Mux/1
  Stbd Thruster Model/3(Torque) -> Mux/3
  Stbd Thruster Model/2(F_sway) -> Mux/2
  Mux1/1 -> Sum/1
  Port Thruster Model/2(F_sway) -> Mux1/2
  Port Thruster Model/1(F_surge) -> Mux1/1
  Port Thruster Model/3(Torque) -> Mux1/3
  Dynamic Model/1(surgeAccel) -> Non-Holonomic Constraint/2(surgeAccel)
  Dynamic Model/2(swayAccel) -> Non-Holonomic Constraint/3(swayAccel)
  Dynamic Model/3(yawAccel) -> Non-Holonomic Constraint/4(YawAccel)
  Y/1 -> Non-Holonomic Constraint/10(Y)
  X/1 -> Non-Holonomic Constraint/9(X)
  Bus Selector/3 -> Non-Holonomic Constraint/7(gyrz)  "<r>"
  Non-Holonomic Constraint/1(NEyaw) -> NEyaw/1
  enabled/1 -> Discrete-Time Integrator1/1
  Discrete-Time Integrator1/1 -> Non-Holonomic Constraint/1(time)
  Nav Messages/1 -> Bus Selector/1
  Bus Selector/4 -> move_part/1(PtThrust)  "<PtThrust>"
  Bus Selector/5 -> move_part/2(PtAzimuth)  "<PtAzimuth>"
  Bus Selector/7 -> move_part/4(StAzimuth)  "<StAzimuth>"
  Bus Selector/6 -> move_part/3(StThrust)  "<StThrust>"
  move_part/1(portMP) -> Port Thruster Model/1(portMP)
  move_part/2(portAzimuth) -> Port Thruster Model/2(portAzimuth)
  move_part/3(stbdMP) -> Stbd Thruster Model/1(stbdMP)
  move_part/4(stbdAzimuth) -> Stbd Thruster Model/2(stbdAzimuth)
  Data Store Read/1 -> move_part/5(noiseLevel)

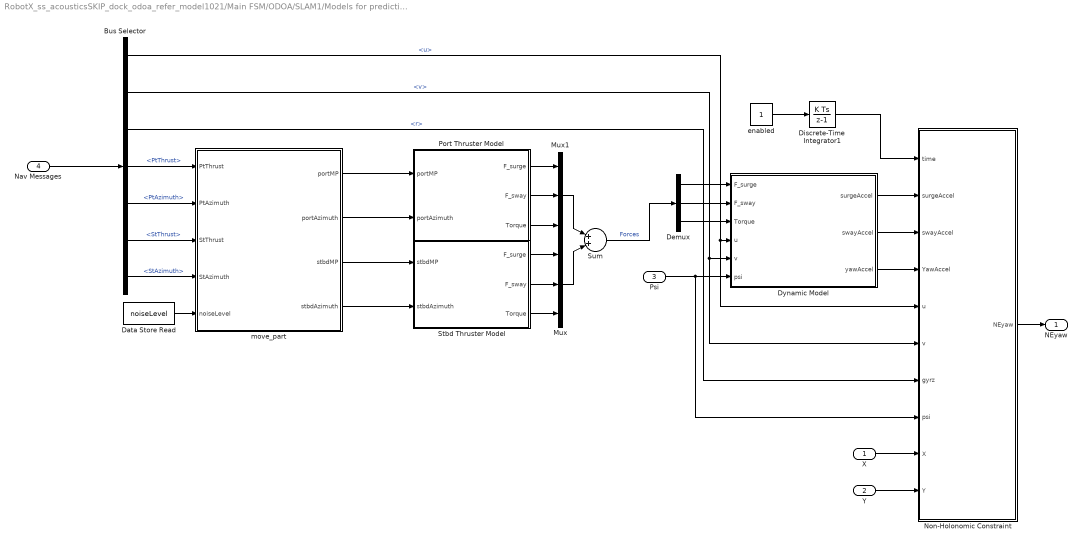
== system RobotX_ss_acousticsSKIP_dock_odoa_refer_model1021/Main FSM/ODOA/SLAM1/Models for prediction/Model12 ==
  X : Inport
  Y : Inport  Port=2
  Psi : Inport  Port=3
  Nav Messages : Inport  Port=4
  Bus Selector : BusSelector  OutputSignals=Velocity.u,Velocity.v,Velocity.r,Port.PtThrust,Port.PtAzimuth,Stbd.StThrust,Stbd.StAzimuth
  Data Store Read : DataStoreRead  DataStoreName=noiseLevel
  Demux : Demux  Outputs=3
  Discrete-Time Integrator1 : DiscreteIntegrator  SampleTime=-1  ICPrevOutput=DiscIntNeverNeededParam  ICPrevScaledInput=DiscIntNeverNeededParam
  Dynamic Model : MATLAB Function  TreatAsAtomicUnit=on
  Mux : Mux  Inputs=3
  Mux1 : Mux  Inputs=3
  Non-Holonomic Constraint : MATLAB Function  TreatAsAtomicUnit=on
  Port Thruster Model : MATLAB Function  TreatAsAtomicUnit=on
  Stbd Thruster Model : MATLAB Function  TreatAsAtomicUnit=on
  Sum : Sum  Inputs=|++|
  enabled : Constant
  move_part : MATLAB Function  TreatAsAtomicUnit=on
  NEyaw : Outport
  wires:
  Sum/1 -> Demux/1  "Forces"
  Bus Selector/2 -> Non-Holonomic Constraint/6(v), Dynamic Model/5(v)  "<v>"
  Bus Selector/1 -> Non-Holonomic Constraint/5(u), Dynamic Model/4(u)  "<u>"
  Psi/1 -> Non-Holonomic Constraint/8(psi), Dynamic Model/6(psi)
  Demux/2 -> Dynamic Model/2(F_sway)
  Demux/3 -> Dynamic Model/3(Torque)
  Demux/1 -> Dynamic Model/1(F_surge)
  Mux/1 -> Sum/2
  Stbd Thruster Model/1(F_surge) -> Mux/1
  Stbd Thruster Model/3(Torque) -> Mux/3
  Stbd Thruster Model/2(F_sway) -> Mux/2
  Mux1/1 -> Sum/1
  Port Thruster Model/2(F_sway) -> Mux1/2
  Port Thruster Model/1(F_surge) -> Mux1/1
  Port Thruster Model/3(Torque) -> Mux1/3
  Dynamic Model/1(surgeAccel) -> Non-Holonomic Constraint/2(surgeAccel)
  Dynamic Model/2(swayAccel) -> Non-Holonomic Constraint/3(swayAccel)
  Dynamic Model/3(yawAccel) -> Non-Holonomic Constraint/4(YawAccel)
  Y/1 -> Non-Holonomic Constraint/10(Y)
  X/1 -> Non-Holonomic Constraint/9(X)
  Bus Selector/3 -> Non-Holonomic Constraint/7(gyrz)  "<r>"
  Non-Holonomic Constraint/1(NEyaw) -> NEyaw/1
  enabled/1 -> Discrete-Time Integrator1/1
  Discrete-Time Integrator1/1 -> Non-Holonomic Constraint/1(time)
  Nav Messages/1 -> Bus Selector/1
  Bus Selector/4 -> move_part/1(PtThrust)  "<PtThrust>"
  Bus Selector/5 -> move_part/2(PtAzimuth)  "<PtAzimuth>"
  Bus Selector/7 -> move_part/4(StAzimuth)  "<StAzimuth>"
  Bus Selector/6 -> move_part/3(StThrust)  "<StThrust>"
  move_part/1(portMP) -> Port Thruster Model/1(portMP)
  move_part/2(portAzimuth) -> Port Thruster Model/2(portAzimuth)
  move_part/3(stbdMP) -> Stbd Thruster Model/1(stbdMP)
  move_part/4(stbdAzimuth) -> Stbd Thruster Model/2(stbdAzimuth)
  Data Store Read/1 -> move_part/5(noiseLevel)

== system RobotX_ss_acousticsSKIP_dock_odoa_refer_model1021/Main FSM/ODOA/SLAM1/Models for prediction/Model13 ==
  X : Inport
  Y : Inport  Port=2
  Psi : Inport  Port=3
  Nav Messages : Inport  Port=4
  Bus Selector : BusSelector  OutputSignals=Velocity.u,Velocity.v,Velocity.r,Port.PtThrust,Port.PtAzimuth,Stbd.StThrust,Stbd.StAzimuth
  Data Store Read : DataStoreRead  DataStoreName=noiseLevel
  Demux : Demux  Outputs=3
  Discrete-Time Integrator1 : DiscreteIntegrator  SampleTime=-1  ICPrevOutput=DiscIntNeverNeededParam  ICPrevScaledInput=DiscIntNeverNeededParam
  Dynamic Model : MATLAB Function  TreatAsAtomicUnit=on
  Mux : Mux  Inputs=3
  Mux1 : Mux  Inputs=3
  Non-Holonomic Constraint : MATLAB Function  TreatAsAtomicUnit=on
  Port Thruster Model : MATLAB Function  TreatAsAtomicUnit=on
  Stbd Thruster Model : MATLAB Function  TreatAsAtomicUnit=on
  Sum : Sum  Inputs=|++|
  enabled : Constant
  move_part : MATLAB Function  TreatAsAtomicUnit=on
  NEyaw : Outport
  wires:
  Sum/1 -> Demux/1  "Forces"
  Bus Selector/2 -> Non-Holonomic Constraint/6(v), Dynamic Model/5(v)  "<v>"
  Bus Selector/1 -> Non-Holonomic Constraint/5(u), Dynamic Model/4(u)  "<u>"
  Psi/1 -> Non-Holonomic Constraint/8(psi), Dynamic Model/6(psi)
  Demux/2 -> Dynamic Model/2(F_sway)
  Demux/3 -> Dynamic Model/3(Torque)
  Demux/1 -> Dynamic Model/1(F_surge)
  Mux/1 -> Sum/2
  Stbd Thruster Model/1(F_surge) -> Mux/1
  Stbd Thruster Model/3(Torque) -> Mux/3
  Stbd Thruster Model/2(F_sway) -> Mux/2
  Mux1/1 -> Sum/1
  Port Thruster Model/2(F_sway) -> Mux1/2
  Port Thruster Model/1(F_surge) -> Mux1/1
  Port Thruster Model/3(Torque) -> Mux1/3
  Dynamic Model/1(surgeAccel) -> Non-Holonomic Constraint/2(surgeAccel)
  Dynamic Model/2(swayAccel) -> Non-Holonomic Constraint/3(swayAccel)
  Dynamic Model/3(yawAccel) -> Non-Holonomic Constraint/4(YawAccel)
  Y/1 -> Non-Holonomic Constraint/10(Y)
  X/1 -> Non-Holonomic Constraint/9(X)
  Bus Selector/3 -> Non-Holonomic Constraint/7(gyrz)  "<r>"
  Non-Holonomic Constraint/1(NEyaw) -> NEyaw/1
  enabled/1 -> Discrete-Time Integrator1/1
  Discrete-Time Integrator1/1 -> Non-Holonomic Constraint/1(time)
  Nav Messages/1 -> Bus Selector/1
  Bus Selector/4 -> move_part/1(PtThrust)  "<PtThrust>"
  Bus Selector/5 -> move_part/2(PtAzimuth)  "<PtAzimuth>"
  Bus Selector/7 -> move_part/4(StAzimuth)  "<StAzimuth>"
  Bus Selector/6 -> move_part/3(StThrust)  "<StThrust>"
  move_part/1(portMP) -> Port Thruster Model/1(portMP)
  move_part/2(portAzimuth) -> Port Thruster Model/2(portAzimuth)
  move_part/3(stbdMP) -> Stbd Thruster Model/1(stbdMP)
  move_part/4(stbdAzimuth) -> Stbd Thruster Model/2(stbdAzimuth)
  Data Store Read/1 -> move_part/5(noiseLevel)

== system RobotX_ss_acousticsSKIP_dock_odoa_refer_model1021/Main FSM/ODOA/SLAM1/Models for prediction/Model14 ==
  X : Inport
  Y : Inport  Port=2
  Psi : Inport  Port=3
  Nav Messages : Inport  Port=4
  Bus Selector : BusSelector  OutputSignals=Velocity.u,Velocity.v,Velocity.r,Port.PtThrust,Port.PtAzimuth,Stbd.StThrust,Stbd.StAzimuth
  Data Store Read : DataStoreRead  DataStoreName=noiseLevel
  Demux : Demux  Outputs=3
  Discrete-Time Integrator1 : DiscreteIntegrator  SampleTime=-1  ICPrevOutput=DiscIntNeverNeededParam  ICPrevScaledInput=DiscIntNeverNeededParam
  Dynamic Model : MATLAB Function  TreatAsAtomicUnit=on
  Mux : Mux  Inputs=3
  Mux1 : Mux  Inputs=3
  Non-Holonomic Constraint : MATLAB Function  TreatAsAtomicUnit=on
  Port Thruster Model : MATLAB Function  TreatAsAtomicUnit=on
  Stbd Thruster Model : MATLAB Function  TreatAsAtomicUnit=on
  Sum : Sum  Inputs=|++|
  enabled : Constant
  move_part : MATLAB Function  TreatAsAtomicUnit=on
  NEyaw : Outport
  wires:
  Sum/1 -> Demux/1  "Forces"
  Bus Selector/2 -> Non-Holonomic Constraint/6(v), Dynamic Model/5(v)  "<v>"
  Bus Selector/1 -> Non-Holonomic Constraint/5(u), Dynamic Model/4(u)  "<u>"
  Psi/1 -> Non-Holonomic Constraint/8(psi), Dynamic Model/6(psi)
  Demux/2 -> Dynamic Model/2(F_sway)
  Demux/3 -> Dynamic Model/3(Torque)
  Demux/1 -> Dynamic Model/1(F_surge)
  Mux/1 -> Sum/2
  Stbd Thruster Model/1(F_surge) -> Mux/1
  Stbd Thruster Model/3(Torque) -> Mux/3
  Stbd Thruster Model/2(F_sway) -> Mux/2
  Mux1/1 -> Sum/1
  Port Thruster Model/2(F_sway) -> Mux1/2
  Port Thruster Model/1(F_surge) -> Mux1/1
  Port Thruster Model/3(Torque) -> Mux1/3
  Dynamic Model/1(surgeAccel) -> Non-Holonomic Constraint/2(surgeAccel)
  Dynamic Model/2(swayAccel) -> Non-Holonomic Constraint/3(swayAccel)
  Dynamic Model/3(yawAccel) -> Non-Holonomic Constraint/4(YawAccel)
  Y/1 -> Non-Holonomic Constraint/10(Y)
  X/1 -> Non-Holonomic Constraint/9(X)
  Bus Selector/3 -> Non-Holonomic Constraint/7(gyrz)  "<r>"
  Non-Holonomic Constraint/1(NEyaw) -> NEyaw/1
  enabled/1 -> Discrete-Time Integrator1/1
  Discrete-Time Integrator1/1 -> Non-Holonomic Constraint/1(time)
  Nav Messages/1 -> Bus Selector/1
  Bus Selector/4 -> move_part/1(PtThrust)  "<PtThrust>"
  Bus Selector/5 -> move_part/2(PtAzimuth)  "<PtAzimuth>"
  Bus Selector/7 -> move_part/4(StAzimuth)  "<StAzimuth>"
  Bus Selector/6 -> move_part/3(StThrust)  "<StThrust>"
  move_part/1(portMP) -> Port Thruster Model/1(portMP)
  move_part/2(portAzimuth) -> Port Thruster Model/2(portAzimuth)
  move_part/3(stbdMP) -> Stbd Thruster Model/1(stbdMP)
  move_part/4(stbdAzimuth) -> Stbd Thruster Model/2(stbdAzimuth)
  Data Store Read/1 -> move_part/5(noiseLevel)

== system RobotX_ss_acousticsSKIP_dock_odoa_refer_model1021/Main FSM/ODOA/SLAM1/Models for prediction/Model15 ==
  X : Inport
  Y : Inport  Port=2
  Psi : Inport  Port=3
  Nav Messages : Inport  Port=4
  Bus Selector : BusSelector  OutputSignals=Velocity.u,Velocity.v,Velocity.r,Port.PtThrust,Port.PtAzimuth,Stbd.StThrust,Stbd.StAzimuth
  Data Store Read : DataStoreRead  DataStoreName=noiseLevel
  Demux : Demux  Outputs=3
  Discrete-Time Integrator1 : DiscreteIntegrator  SampleTime=-1  ICPrevOutput=DiscIntNeverNeededParam  ICPrevScaledInput=DiscIntNeverNeededParam
  Dynamic Model : MATLAB Function  TreatAsAtomicUnit=on
  Mux : Mux  Inputs=3
  Mux1 : Mux  Inputs=3
  Non-Holonomic Constraint : MATLAB Function  TreatAsAtomicUnit=on
  Port Thruster Model : MATLAB Function  TreatAsAtomicUnit=on
  Stbd Thruster Model : MATLAB Function  TreatAsAtomicUnit=on
  Sum : Sum  Inputs=|++|
  enabled : Constant
  move_part : MATLAB Function  TreatAsAtomicUnit=on
  NEyaw : Outport
  wires:
  Sum/1 -> Demux/1  "Forces"
  Bus Selector/2 -> Non-Holonomic Constraint/6(v), Dynamic Model/5(v)  "<v>"
  Bus Selector/1 -> Non-Holonomic Constraint/5(u), Dynamic Model/4(u)  "<u>"
  Psi/1 -> Non-Holonomic Constraint/8(psi), Dynamic Model/6(psi)
  Demux/2 -> Dynamic Model/2(F_sway)
  Demux/3 -> Dynamic Model/3(Torque)
  Demux/1 -> Dynamic Model/1(F_surge)
  Mux/1 -> Sum/2
  Stbd Thruster Model/1(F_surge) -> Mux/1
  Stbd Thruster Model/3(Torque) -> Mux/3
  Stbd Thruster Model/2(F_sway) -> Mux/2
  Mux1/1 -> Sum/1
  Port Thruster Model/2(F_sway) -> Mux1/2
  Port Thruster Model/1(F_surge) -> Mux1/1
  Port Thruster Model/3(Torque) -> Mux1/3
  Dynamic Model/1(surgeAccel) -> Non-Holonomic Constraint/2(surgeAccel)
  Dynamic Model/2(swayAccel) -> Non-Holonomic Constraint/3(swayAccel)
  Dynamic Model/3(yawAccel) -> Non-Holonomic Constraint/4(YawAccel)
  Y/1 -> Non-Holonomic Constraint/10(Y)
  X/1 -> Non-Holonomic Constraint/9(X)
  Bus Selector/3 -> Non-Holonomic Constraint/7(gyrz)  "<r>"
  Non-Holonomic Constraint/1(NEyaw) -> NEyaw/1
  enabled/1 -> Discrete-Time Integrator1/1
  Discrete-Time Integrator1/1 -> Non-Holonomic Constraint/1(time)
  Nav Messages/1 -> Bus Selector/1
  Bus Selector/4 -> move_part/1(PtThrust)  "<PtThrust>"
  Bus Selector/5 -> move_part/2(PtAzimuth)  "<PtAzimuth>"
  Bus Selector/7 -> move_part/4(StAzimuth)  "<StAzimuth>"
  Bus Selector/6 -> move_part/3(StThrust)  "<StThrust>"
  move_part/1(portMP) -> Port Thruster Model/1(portMP)
  move_part/2(portAzimuth) -> Port Thruster Model/2(portAzimuth)
  move_part/3(stbdMP) -> Stbd Thruster Model/1(stbdMP)
  move_part/4(stbdAzimuth) -> Stbd Thruster Model/2(stbdAzimuth)
  Data Store Read/1 -> move_part/5(noiseLevel)

== system RobotX_ss_acousticsSKIP_dock_odoa_refer_model1021/Main FSM/ODOA/SLAM1/Models for prediction/Model16 ==
  X : Inport
  Y : Inport  Port=2
  Psi : Inport  Port=3
  Nav Messages : Inport  Port=4
  Bus Selector : BusSelector  OutputSignals=Velocity.u,Velocity.v,Velocity.r,Port.PtThrust,Port.PtAzimuth,Stbd.StThrust,Stbd.StAzimuth
  Data Store Read : DataStoreRead  DataStoreName=noiseLevel
  Demux : Demux  Outputs=3
  Discrete-Time Integrator1 : DiscreteIntegrator  SampleTime=-1  ICPrevOutput=DiscIntNeverNeededParam  ICPrevScaledInput=DiscIntNeverNeededParam
  Dynamic Model : MATLAB Function  TreatAsAtomicUnit=on
  Mux : Mux  Inputs=3
  Mux1 : Mux  Inputs=3
  Non-Holonomic Constraint : MATLAB Function  TreatAsAtomicUnit=on
  Port Thruster Model : MATLAB Function  TreatAsAtomicUnit=on
  Stbd Thruster Model : MATLAB Function  TreatAsAtomicUnit=on
  Sum : Sum  Inputs=|++|
  enabled : Constant
  move_part : MATLAB Function  TreatAsAtomicUnit=on
  NEyaw : Outport
  wires:
  Sum/1 -> Demux/1  "Forces"
  Bus Selector/2 -> Non-Holonomic Constraint/6(v), Dynamic Model/5(v)  "<v>"
  Bus Selector/1 -> Non-Holonomic Constraint/5(u), Dynamic Model/4(u)  "<u>"
  Psi/1 -> Non-Holonomic Constraint/8(psi), Dynamic Model/6(psi)
  Demux/2 -> Dynamic Model/2(F_sway)
  Demux/3 -> Dynamic Model/3(Torque)
  Demux/1 -> Dynamic Model/1(F_surge)
  Mux/1 -> Sum/2
  Stbd Thruster Model/1(F_surge) -> Mux/1
  Stbd Thruster Model/3(Torque) -> Mux/3
  Stbd Thruster Model/2(F_sway) -> Mux/2
  Mux1/1 -> Sum/1
  Port Thruster Model/2(F_sway) -> Mux1/2
  Port Thruster Model/1(F_surge) -> Mux1/1
  Port Thruster Model/3(Torque) -> Mux1/3
  Dynamic Model/1(surgeAccel) -> Non-Holonomic Constraint/2(surgeAccel)
  Dynamic Model/2(swayAccel) -> Non-Holonomic Constraint/3(swayAccel)
  Dynamic Model/3(yawAccel) -> Non-Holonomic Constraint/4(YawAccel)
  Y/1 -> Non-Holonomic Constraint/10(Y)
  X/1 -> Non-Holonomic Constraint/9(X)
  Bus Selector/3 -> Non-Holonomic Constraint/7(gyrz)  "<r>"
  Non-Holonomic Constraint/1(NEyaw) -> NEyaw/1
  enabled/1 -> Discrete-Time Integrator1/1
  Discrete-Time Integrator1/1 -> Non-Holonomic Constraint/1(time)
  Nav Messages/1 -> Bus Selector/1
  Bus Selector/4 -> move_part/1(PtThrust)  "<PtThrust>"
  Bus Selector/5 -> move_part/2(PtAzimuth)  "<PtAzimuth>"
  Bus Selector/7 -> move_part/4(StAzimuth)  "<StAzimuth>"
  Bus Selector/6 -> move_part/3(StThrust)  "<StThrust>"
  move_part/1(portMP) -> Port Thruster Model/1(portMP)
  move_part/2(portAzimuth) -> Port Thruster Model/2(portAzimuth)
  move_part/3(stbdMP) -> Stbd Thruster Model/1(stbdMP)
  move_part/4(stbdAzimuth) -> Stbd Thruster Model/2(stbdAzimuth)
  Data Store Read/1 -> move_part/5(noiseLevel)
